simulink model "Three_Phase_VSI_with_VF_Control_of_Induction_Motors"  (R2025a)
settings: Solver=ode23tb  StartTime=0.0  StopTime=5  MaxStep=1e-4  RelTol=1e-3
libraries: spsIGBTDiodeLib x6, spsSawtoothGeneratorLib x3, simulink x2, spsAsynchronousMachineSIUnitsLib x1, spsVoltageMeasurementLib x1, spsDCVoltageSourceLib x1, sps_lib x1
settings Model: Creator=Jawad  LastModifiedBy=Jawad

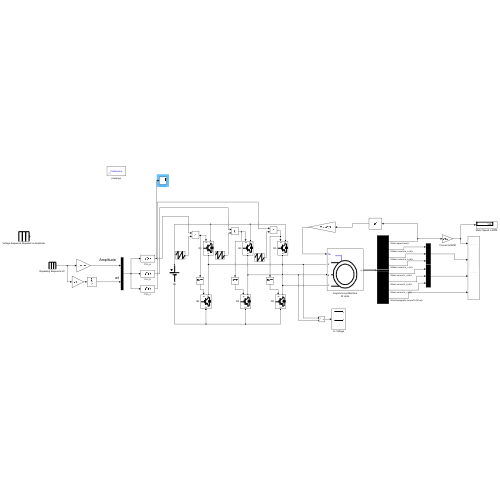
[thumbnail: Simulink's stored preview of the top-level diagram]
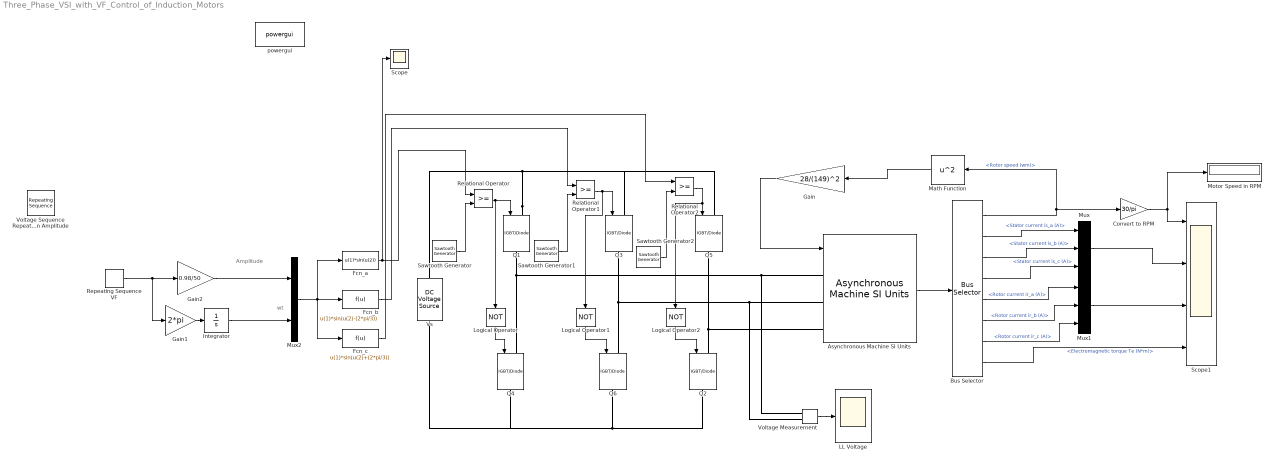
== system Three_Phase_VSI_with_VF_Control_of_Induction_Motors ==
  note: Amplitude
  note: wt
  Asynchronous Machine SI Units : spsAsynchronousMachineSIUnitsLib/Asynchronous Machine SI Units  RotorType=Squirrel-cage  PresetModel="15:  5.4 HP (4KW)   400 V  50Hz 1430 RPM"  MechanicalLoad=Torque Tm  ShowDetailedParameters=on  ReferenceFrame=Rotor  Units=SI  MeasurementBus=off  NominalParameters=[4000 400 50]  VoltageRatio=1  Stator=[1.405 0.005839]  Rotor=[1.395 0.005839]  Cage1=[0.4155 0.002066]  Cage2=[0.4168 0.0003495]  Lm=0.1722  Mechanical=[0.0131 0.002985 2]  PolePairs=2  InitialConditions=[1 0 0 0 0 0 0 0]  SimulateSaturation=off  Saturation=[14.03593122, 27.81365428, 53.79336849, 72.68890987, 97.98006896, 148.6815601, 215.7428561, 302.9841135, 428.7778367 ; 230, 322, 414, 460, 506, 552, 598, 644, 690]  LoadFlowParameters=1492000  TsPowergui=0  TsBlock=-1  IterativeModel=Trapezoidal non iterative  IterativeDiscreteModel=Trapezoidal non iterative  Pmec=1.492e+006
  Bus Selector : BusSelector  OutputSignals=Mechanical.Rotor speed (wm),Stator measurements.Stator current is_a (A),Stator measurements.Stator current is_b (A),Stator measurements.Stator current is_c (A),Rotor measurements.Rotor current ir_a (A),Rotor measurements.Rotor current ir_b (A),Rotor measurements.Rotor current ir_c (A),Mechanical.Electromagnetic torque Te (N*m)
  Convert to RPM : Gain  Gain=30/pi
  Fcn_a : Fcn  Expr=u(1)*sin(u(2))
  Fcn_b : Fcn  Expr=u(1)*sin(u(2)-(2*pi/3))
  Fcn_c : Fcn  Expr=u(1)*sin(u(2)+(2*pi/3))
  Gain : Gain  Gain=28/(149)^2
  Gain1 : Gain  Gain=2*pi
  Gain2 : Gain  Gain=0.98/50
  Integrator : Integrator
  LL Voltage : Scope
      settings: ActiveDisplayYMinimum=-812.5330426089522  ActiveDisplayYMaximum=812.53862765807014
  Logical Operator : Logic  Operator=NOT  AllPortsSameDT=off  OutDataTypeStr=boolean
  Logical Operator1 : Logic  Operator=NOT  AllPortsSameDT=off  OutDataTypeStr=boolean
  Logical Operator2 : Logic  Operator=NOT  AllPortsSameDT=off  OutDataTypeStr=boolean
  Math Function : Math  Operator=square
  Motor Speed in RPM : Display
  Mux : Mux  Inputs=3
  Mux1 : Mux  Inputs=3
  Mux2 : Mux  Inputs=2
  Q{1..6} (6 alike) : spsIGBTDiodeLib/IGBT//Diode  Ron=1e-3  Rs=1e5  Cs=inf  Measurements=off
  Relational Operator : RelationalOperator  OutDataTypeStr=boolean  RndMeth=Simplest  InputSameDT=off
  Relational Operator1 : RelationalOperator  OutDataTypeStr=boolean  RndMeth=Simplest  InputSameDT=off
  Relational Operator2 : RelationalOperator  OutDataTypeStr=boolean  RndMeth=Simplest  InputSameDT=off
  Repeating Sequence VF : simulink/Sources/Repeating Sequence  rep_seq_t=[0 0.2 10]  rep_seq_y=[0 50 50]
  Sawtooth Generator : spsSawtoothGeneratorLib/Sawtooth Generator  Freq=1000  Phase=180  Ts=0
  Sawtooth Generator1 : spsSawtoothGeneratorLib/Sawtooth Generator  Freq=1000  Phase=180  Ts=0
  Sawtooth Generator2 : spsSawtoothGeneratorLib/Sawtooth Generator  Freq=1000  Phase=180  Ts=0
  Scope : Scope
      settings: ActiveDisplayYMinimum=-1.225  ActiveDisplayYMaximum=1.225  DataLoggingVariableName=ScopeData2
  Scope1 : Scope  NumInputPorts=4
      settings: ActiveDisplayString=4  Title=Electromagnetic Torque  ActiveDisplayYMinimum=-81.1027319727876  ActiveDisplayYMaximum=169.27348685426449
  Voltage Measurement : spsVoltageMeasurementLib/Voltage Measurement  PhasorSimulation=off  OutputType=Complex  PSBequivalent=0
  Voltage Sequence Repeater in Amplitude : simulink/Sources/Repeating Sequence  rep_seq_t=[0 0.2 10]  rep_seq_y=[0 327 327]
  Vs : spsDCVoltageSourceLib/DC Voltage Source  Amplitude=650  Measurements=None
  powergui : sps_lib/powergui  Priority=1  SimulationMode=Continuous  SampleTime=50e-6  frequency=60  Iterations=50  frequencyindice=50  Pbase=100e6  ErrMax=1e-4  UnitsV=kV  UnitsW=MW  buscounter=0  FunctionMessages=off  echomessages=off  EnableUseOfTLC=off  CurrentSourceSwitches=off  DisableSnubberDevices=off  DisableRonSwitches=off  DisableVfSwitches=off  DisplayEquations=off  AutomaticDiscreteSolvers=off  SolverType=Tustin/Backward Euler (TBE)  Interpol=off  ExternalGateDelay=off  methode=off  Ts=100  x0status=blocks  SPID=on  SwTol=0  HookPort=off  NonlinearTolerance=1e-4  nMaxIteration=100  ContinueOnMaxIteration=off  RestoreLinks=warning  ResistiveCurrentMeasurement=off  Frange=[0:2:500]  Ylog=off  Xlog=on  ShowGrid=off  save=off  variable=ZData  structure=0  ZoomFFT=off  StartTime=0.0  cycles=1  DisplayStyle=1  fundamental=60  FreqAxis=off  MaxFrequency=1000  frequencyindicesteady=1  RmsSteady=1  display=off
  wires:
  Bus Selector/8 -> Scope1/4  "<Electromagnetic torque Te (N*m)>"
  Bus Selector/3 -> Mux/2  "<Stator current is_b (A)>"
  Bus Selector/7 -> Mux1/3  "<Rotor current ir_c (A)>"
  Bus Selector/4 -> Mux/3  "<Stator current is_c (A)>"
  Asynchronous Machine SI Units/1 -> Bus Selector/1
  Bus Selector/1 -> Math Function/1, Convert to RPM/1  "<Rotor speed (wm)>"
  Bus Selector/6 -> Mux1/2  "<Rotor current ir_b (A)>"
  Convert to RPM/1 -> Scope1/1, Motor Speed in RPM/1
  Mux/1 -> Scope1/2
  Bus Selector/2 -> Mux/1  "<Stator current is_a (A)>"
  Math Function/1 -> Gain/1
  Mux1/1 -> Scope1/3
  Bus Selector/5 -> Mux1/1  "<Rotor current ir_a (A)>"
  Mux2/1 -> Fcn_c/1, Fcn_b/1, Fcn_a/1
  Repeating Sequence VF/1 -> Gain2/1, Gain1/1
  Gain1/1 -> Integrator/1
  Integrator/1 -> Mux2/2
  Logical Operator1/1 -> Q6/1
  Logical Operator2/1 -> Q2/1
  Sawtooth Generator2/1 -> Relational Operator2/2
  Relational Operator2/1 -> Logical Operator2/1, Q5/1
  Sawtooth Generator1/1 -> Relational Operator1/2
  Sawtooth Generator/1 -> Relational Operator/2
  Relational Operator1/1 -> Logical Operator1/1, Q3/1
  Relational Operator/1 -> Q1/1, Logical Operator/1
  Logical Operator/1 -> Q4/1
  Fcn_a/1 -> Scope/1, Relational Operator/1
  Fcn_b/1 -> Relational Operator1/1
  Fcn_c/1 -> Relational Operator2/1
  Voltage Measurement/1 -> LL Voltage/1
  Gain/1 -> Asynchronous Machine SI Units/1
  Gain2/1 -> Mux2/1
  connections:
  Q1/LConn1 -- Q5/LConn1 -- Q3/LConn1 -- Vs/RConn1
  Q6/RConn1 -- Q2/RConn1 -- Q4/RConn1 -- Vs/LConn1
  Q6/LConn1 -- Q3/RConn1 -- Voltage Measurement/LConn2 -- Asynchronous Machine SI Units/LConn2
  Q4/LConn1 -- Voltage Measurement/LConn1 -- Asynchronous Machine SI Units/LConn1 -- Q1/RConn1
  Q2/LConn1 -- Q5/RConn1 -- Asynchronous Machine SI Units/LConn3
